simulink model "s573a"  (Simulink 5.1)
settings: Solver=ode45  StartTime=0.0  StopTime=100.0  RelTol=1e-3
libraries: simulink x1
settings Model: LastModifiedBy=user_father  BooleanDataType=on  ProdHWDeviceType=Microprocessor

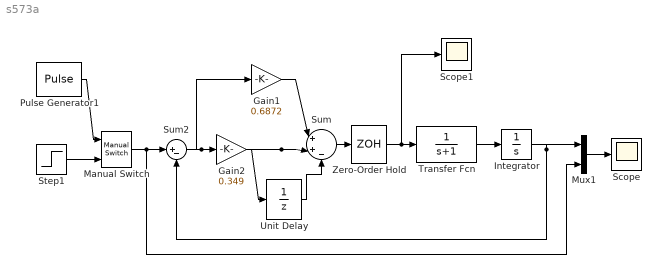
== system s573a ==
  Gain1 : Gain  Gain=0.6872  SaturateOnIntegerOverflow=on
  Gain2 : Gain  Gain=0.349  SaturateOnIntegerOverflow=on
  Integrator : Integrator
  Manual Switch : simulink/Signal Routing/Manual Switch  sw=0  action=0
  Mux1 : Mux  Inputs=2
  Pulse Generator1 : DiscretePulseGenerator  PulseType=Time based  Period=60  PulseWidth=50
  Scope : Scope
  Scope1 : Scope
  Step1 : Step  Time=0  SampleTime=0
  Sum : Sum  Inputs=|++-  SaturateOnIntegerOverflow=on
  Sum2 : Sum  Inputs=|+-  SaturateOnIntegerOverflow=on
  Transfer Fcn : TransferFcn  Denominator=[1 1]
  Unit Delay : UnitDelay
  Zero-Order Hold : ZeroOrderHold
  wires:
  Mux1/1 -> Scope/1
  Pulse Generator1/1 -> Manual Switch/1
  Manual Switch/1 -> Sum2/1, Mux1/2
  Step1/1 -> Manual Switch/2
  Sum2/1 -> Gain1/1, Gain2/1
  Gain1/1 -> Sum/1
  Gain2/1 -> Sum/2, Unit Delay/1
  Unit Delay/1 -> Sum/3
  Transfer Fcn/1 -> Integrator/1
  Integrator/1 -> Mux1/1, Sum2/2
  Sum/1 -> Zero-Order Hold/1
  Zero-Order Hold/1 -> Transfer Fcn/1, Scope1/1
